simulink model "Main_simulation_gio"  (R2021b)
settings: Solver=FixedStepAuto  StartTime=0.0  StopTime=Time  FixedStep=0.1  RelTol=1e-13  AbsTol=1e-19
values from neighbouring files (symbols this model uses):
  a = 8.6251e06    (= 8625100)    [main_code.m]
  A_BN_0 = eye(3)    [main_code.m]
  A_rw = [1 0 0 1/sqrt(3);         0 1 0 1/sqrt(3) ... (first row only)    [main_code.m]
  A_rw_star = [5/6 -1/6 -1/6;              -1/6  5/6 -1/6 ... (first row only)    [main_code.m]
  c = 2.99792*10^8    (= 299792000)    [main_code.m]
  e = 0.1195    [main_code.m]
  G = [gn, gm, gvali, gsvi]    [main_code.m]
  H = [hn, hm, hvali, hsvi]    [main_code.m]
  i = 0.3815    [main_code.m]
  MB = [1; 0.3; 0.3; 0.3]    [main_code.m]
  mr = 1.2*1e-4    (= 0.00012)    [main_code.m]
  mu_P = G * Mt    (= 398527110340000)    [main_code.m]
  omega_0 = [w_0x; w_0y; w_0z]    [main_code.m]
  p_acc = 0.5    [main_code.m]
  rho_d_MB = 0.1    [main_code.m]
  rho_d_SP = 0.1    [main_code.m]
  rho_s_MB = 0.5    [main_code.m]
  rho_s_SP = 0.1    [main_code.m]
  sig_b = sig_b^2    [main_code.m]
  sig_n = 0.15*pi/180/3600/sqrt(t_sample)    [main_code.m]
  SP = [3; 0.3; 1; 0.1]    [main_code.m]
  T = 2*pi / n    [main_code.m]
  t_sample = 1    [main_code.m]
  theta_0 = 0    [main_code.m]
undefined symbols (not defined in the file or in its folder): magnitude, theta0
libraries: matrix_library x13, vrlib x7, simulink x3, simulink_extras x1
(part 5 of 5)

== system Main_simulation_gio/Sensors/Magnetometer1/Magnetometer /Error Matrices/A_NonOrtho ==
  Constant : Constant
  Constant1 : Constant  Value=0
  Constant2 : Constant  Value=0
  Constant3 : Constant  Value=-0.04
  Constant4 : Constant
  Constant5 : Constant  Value=0
  Constant6 : Constant  Value=0.02
  Constant7 : Constant  Value=0.01
  Constant8 : Constant
  Reshape : Reshape  OutputDimensionality=Customize  OutputDimensions=[3,3]
  Vector Concatenate : Concatenate  NumInputs=9
  A_no : Outport
  wires:
  [A31] -> Vector Concatenate/3
  [A12] -> Vector Concatenate/4
  [A21] -> Vector Concatenate/2
  [A33] -> Vector Concatenate/9
  [A32] -> Vector Concatenate/6
  [A22] -> Vector Concatenate/5
  [A13] -> Vector Concatenate/7
  [A23] -> Vector Concatenate/8
  [A11] -> Vector Concatenate/1
  Vector Concatenate/1 -> Reshape/1
  Reshape/1 -> A_no/1
  Constant/1 -> [A11]
  Constant1/1 -> [A21]
  Constant2/1 -> [A31]
  Constant3/1 -> [A12]
  Constant4/1 -> [A22]
  Constant5/1 -> [A32]
  Constant6/1 -> [A13]
  Constant7/1 -> [A23]
  Constant8/1 -> [A33]

== system Main_simulation_gio/Sensors/Magnetometer1/Magnetometer /Error Matrices/A_ScaleFactor ==
  Constant : Constant  Value=1.08
  Constant{1..2,4..7} (6 alike) : Constant  Value=0
  Constant3 : Constant  Value=0.95
  Constant8 : Constant  Value=1.10
  Reshape : Reshape  OutputDimensionality=Customize  OutputDimensions=[3,3]
  Vector Concatenate : Concatenate  NumInputs=9
  A_sf : Outport
  wires:
  [A31] -> Vector Concatenate/3
  [A12] -> Vector Concatenate/4
  [A21] -> Vector Concatenate/2
  [A33] -> Vector Concatenate/9
  [A32] -> Vector Concatenate/6
  [A22] -> Vector Concatenate/5
  [A13] -> Vector Concatenate/7
  [A23] -> Vector Concatenate/8
  [A11] -> Vector Concatenate/1
  Vector Concatenate/1 -> Reshape/1
  Reshape/1 -> A_sf/1
  Constant/1 -> [A11]
  Constant1/1 -> [A21]
  Constant2/1 -> [A31]
  Constant4/1 -> [A12]
  Constant3/1 -> [A22]
  Constant5/1 -> [A32]
  Constant6/1 -> [A13]
  Constant7/1 -> [A23]
  Constant8/1 -> [A33]

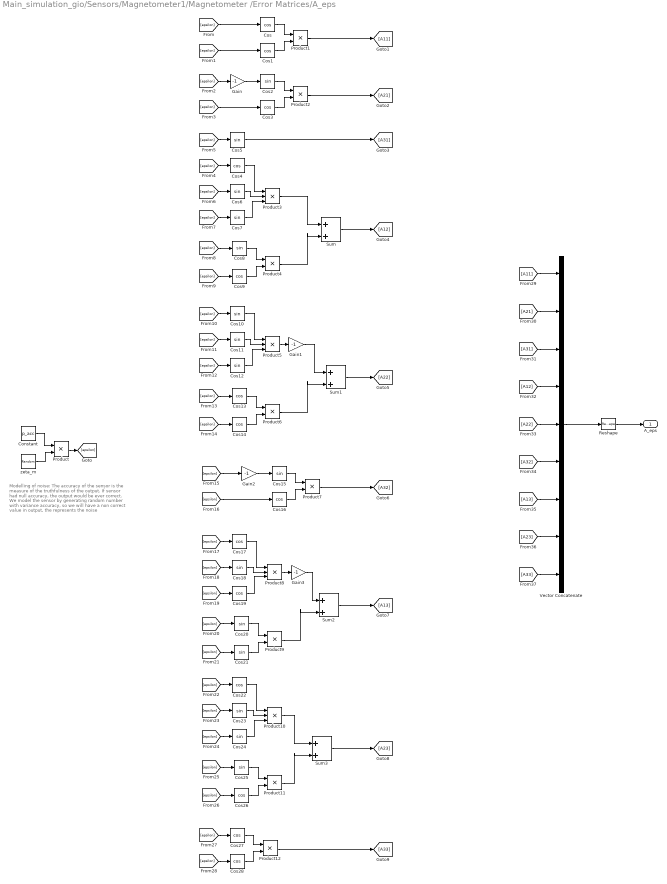
== system Main_simulation_gio/Sensors/Magnetometer1/Magnetometer /Error Matrices/A_eps ==
  note: Modelling of noise: The accuracy of the sensor
      | is the measure of the truthfulness of the output.
      | If sensor had null accuracy, the output would be
      | ever correct. We model the  sensor by generating
      | random number with variance accuracy, so we
      | will have a non correct value in output, the
      | represents the noise
  Constant : Constant  Value=p_acc
  Cos{,1,3..4,9,13..14,16..17,19,22,26..28} (14 alike) : Trigonometry  Operator=cos
  Cos{2,5..8,10..12,15,18,20..21,23..25} (15 alike) : Trigonometry
  Gain{,1..3} (4 alike) : Gain  Gain=-1
  Product{,1..2,4,6..7,9,11..12} (9 alike) : Product
  Product{3,5,8,10} (4 alike) : Product  Inputs=3
  Reshape : Reshape  OutputDimensionality=Customize  OutputDimensions=[3,3]
  Sum{,1..3} (4 alike) : Sum  Inputs=|+|+|
  Vector Concatenate : Concatenate  NumInputs=9
  zeta_m : RandomNumber  Variance=p_acc  Seed=1  SampleTime=t_sample
  A_eps : Outport
  wires:
  Reshape/1 -> A_eps/1
  Vector Concatenate/1 -> Reshape/1
  Constant/1 -> Product/1
  zeta_m/1 -> Product/2
  Product/1 -> [epsilon]
  [epsilon] -> Cos/1
  [epsilon] -> Cos1/1
  Cos/1 -> Product1/1
  Cos1/1 -> Product1/2
  Product1/1 -> [A11]
  Cos2/1 -> Product2/1
  Cos3/1 -> Product2/2
  [epsilon] -> Cos3/1
  Product2/1 -> [A21]
  [epsilon] -> Gain/1
  Gain/1 -> Cos2/1
  [epsilon] -> Cos5/1
  Cos5/1 -> [A31]
  Cos4/1 -> Product3/1
  Cos6/1 -> Product3/2
  [epsilon] -> Cos4/1
  [epsilon] -> Cos6/1
  Product3/1 -> Sum/1
  [epsilon] -> Cos7/1
  Cos7/1 -> Product3/3
  [epsilon] -> Cos8/1
  Product4/1 -> Sum/2
  [epsilon] -> Cos9/1
  Cos9/1 -> Product4/2
  Cos8/1 -> Product4/1
  Sum/1 -> [A12]
  [epsilon] -> Cos11/1
  [epsilon] -> Cos10/1
  Cos11/1 -> Product5/2
  Cos10/1 -> Product5/1
  [epsilon] -> Cos13/1
  Sum1/1 -> [A22]
  Cos13/1 -> Product6/1
  [epsilon] -> Cos14/1
  Cos12/1 -> Product5/3
  Cos14/1 -> Product6/2
  Product6/1 -> Sum1/2
  [epsilon] -> Cos12/1
  Product5/1 -> Gain1/1
  Gain1/1 -> Sum1/1
  Gain2/1 -> Cos15/1
  [epsilon] -> Gain2/1
  Product7/1 -> [A32]
  Cos16/1 -> Product7/2
  Cos15/1 -> Product7/1
  [epsilon] -> Cos16/1
  Gain3/1 -> Sum2/1
  Product8/1 -> Gain3/1
  Cos18/1 -> Product8/2
  [epsilon] -> Cos18/1
  Sum2/1 -> [A13]
  Cos20/1 -> Product9/1
  Cos17/1 -> Product8/1
  [epsilon] -> Cos19/1
  Cos19/1 -> Product8/3
  Product9/1 -> Sum2/2
  [epsilon] -> Cos17/1
  Cos21/1 -> Product9/2
  [epsilon] -> Cos20/1
  [epsilon] -> Cos21/1
  [epsilon] -> Cos23/1
  [epsilon] -> Cos22/1
  Cos23/1 -> Product10/2
  Cos22/1 -> Product10/1
  [epsilon] -> Cos25/1
  Sum3/1 -> [A23]
  Cos25/1 -> Product11/1
  [epsilon] -> Cos26/1
  Product10/1 -> Sum3/1
  Cos24/1 -> Product10/3
  Cos26/1 -> Product11/2
  Product11/1 -> Sum3/2
  [epsilon] -> Cos24/1
  Cos27/1 -> Product12/1
  Cos28/1 -> Product12/2
  [epsilon] -> Cos27/1
  [epsilon] -> Cos28/1
  Product12/1 -> [A33]
  [A11] -> Vector Concatenate/1
  [A21] -> Vector Concatenate/2
  [A31] -> Vector Concatenate/3
  [A12] -> Vector Concatenate/4
  [A22] -> Vector Concatenate/5
  [A32] -> Vector Concatenate/6
  [A13] -> Vector Concatenate/7
  [A23] -> Vector Concatenate/8
  [A33] -> Vector Concatenate/9

== system Main_simulation_gio/Sensors/Magnetometer1/b_B computation/Saturation/If Action Subsystem ==
  b_B : Inport
  Action Port : ActionPort  ActionPortLabel=if(u1 < mr)
  b_B* : Outport
  wires:
  b_B/1 -> b_B*/1

== system Main_simulation_gio/Sensors/Magnetometer1/b_B computation/Saturation/If Action Subsystem1 ==
  mr : Inport
  b_B : Inport  Port=2
  Action Port : ActionPort  ActionPortLabel=else
  Normalize Vector : vrlib/Utilities/Normalize Vector  maxzero=0
  Product : Product
  b_B_sat : Outport
  wires:
  b_B/1 -> Normalize Vector/1
  Product/1 -> b_B_sat/1
  mr/1 -> Product/1
  Normalize Vector/1 -> Product/2

== matlab function Main_simulation_gio/Attitude determination/MATLAB Function ==
  data: K input; V output; D output
function [V, D] = fcn(K)
[V,D] = eig(K);
end

== matlab function Main_simulation_gio/Enviroment/Magnetic field/b_B/MATLAB Function ==
  data: r_LVLH input; r input; b_N output; t input; G input; H input
function b_N  = magnet(r_LVLH, r, t, G, H)
% Inputs
% r Geocentric radius
% theta Latitude measured in degrees positive from equator
% phi Longitude measured in degrees positive east from Greenwich
%
% Outputs - magnetic field strength in local tangential coordinates
% Br B in radial direction
% Bt B in theta direction
% Bp B in phi direction

% Computing the right ascension alpha, the declination delta, the longitude lon and the co-latitude phi
r_norm = norm(r_LVLH);
delta = asin(r_LVLH(3)/r_norm);
if(r_LVLH(2)/r_norm > 0)
    alpha = acos((r_LVLH(1)/r_norm)/cos(delta));
else 
    alpha = 2*pi -  acos((r_LVLH(1)/r_norm)/cos(delta));
end
theta = -delta;
om_E = deg2rad(15.04)/3600;
Gren_lon = om_E*t;
phi = (alpha - Gren_lon);

% Checks to see if located at either pole to avoid singularities
if (theta>-0.00000001 && theta<0.00000001)
theta=0.00000001;
elseif(theta<180.00000001 && theta>179.99999999)
theta=179.99999999;
end
% The angles must be converted from degrees into radians
theta=(90-theta)*pi/180;
phi = phi*pi/180;
a=6371.2; % Reference radius used in IGRF
% This section of the code simply reads in the g and h Schmidt
% quasi-normalized coefficients
gn = G(:,1);
gm = G(:,2);
gvali = G(:,3);
hn = H(:,1);
hm = H(:,2);
hvali = H(:,3);
%[gn, gm, gvali, ~] = textread('igrfSg.txt','%f %f %f %f');
%[hn, hm, hvali, ~]= textread('igrfSh.txt','%f %f %f %f');
N=max(gn);
g=zeros(N,N+1);
h=zeros(N,N+1);
for x=1:length(gn)
g(gn(x),gm(x)+1) = gvali(x);
h(hn(x),hm(x)+1) = hvali(x);
end
% Initialize each of the variables
% Br B in the radial driection
% Bt B in the theta direction
% Bp B in the phi direction
% P The associated Legendre polynomial evaluated at cos(theta)
% The nomenclature for the recursive values generally follows
% the form P10 = P(n-1,m-0)
% dP The partial derivative of P with respect to theta
Br=0; Bt=0; Bp=0;
P11=1; P10=P11;
dP11=0; dP10=dP11;
for m=0:N
for n=1:N
if m<=n
% Calculate Legendre polynomials and derivatives recursively
if n==m
P2 = sin(theta)*P11;
dP2 = sin(theta)*dP11 + cos(theta)*P11;
P11=P2; P10=P11; P20=0;
dP11=dP2; dP10=dP11; dP20=0;
elseif n==1
P2 = cos(theta)*P10;
dP2 = cos(theta)*dP10 - sin(theta)*P10;
P20=P10; P10=P2;
dP20=dP10; dP10=dP2;
else
P20=P10;
dP20=dP10;
K = ((n-1)^2-m^2)/((2*n-1)*(2*n-3));
P2 = cos(theta)*P10 - K*P20;
dP2 = cos(theta)*dP10 - sin(theta)*P10 - K*dP20;
P10=P2;
dP10=dP2;
end
% Calculate Br, Bt, and Bp
Br = Br + (a/r)^(n+2)*(n+1)*...
((g(n,m+1)*cos(m*phi) + h(n,m+1)*sin(m*phi))*P2);
Bt = Bt + (a/r)^(n+2)*...
((g(n,m+1)*cos(m*phi) + h(n,m+1)*sin(m*phi))*dP2);
Bp = Bp + (a/r)^(n+2)*...
(m*(-g(n,m+1)*sin(m*phi) + h(n,m+1)*cos(m*phi))* P2);
end
end
end
% Spherical coordinates
Br = Br;
Bt = -Bt;
Bp = -Bp / sin(theta);

% Inertial cartesian coordinates
LST = Gren_lon + phi;
lat = theta;
Bx = (Br*cos(lat)+Bt*sin(lat))*cos(LST) - Bp*sin(LST);
By = (Br*cos(lat)+Bt*sin(lat))*sin(LST) + Bp*cos(LST);
Bz = (Br*sin(lat)+Bt*cos(lat));

b_N = [Bx; By; Bz];

end

== matlab function Main_simulation_gio/Inertia matrix/MATLAB Function ==
  data: u input; V output; D output
function [V,D] = fcn(u)

[V,D] = eig(u);
end
